simulink model "HostSerial_Receive"  (R2023b)
settings: Solver=FixedStepAuto  StartTime=0.0  StopTime=inf  FixedStep=0.001  RelTol=1e-3
libraries: instrumentseriallib x2
settings Model: Creator=ADMIN  LastModifiedBy=ADMIN
settings DataIOCC: ReturnWorkspaceOutputs=off
settings DebuggingCC: ParameterPrecisionLossMsg=none

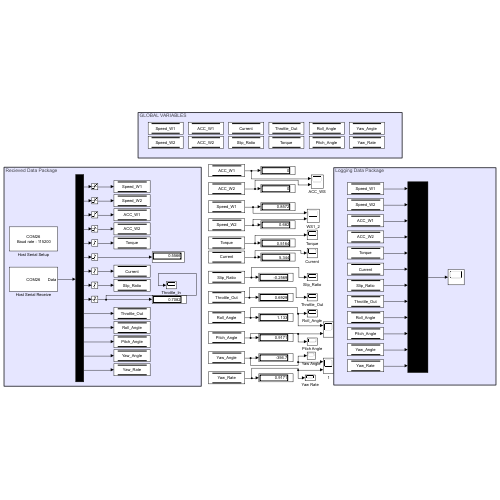
[thumbnail: Simulink's stored preview of the top-level diagram]
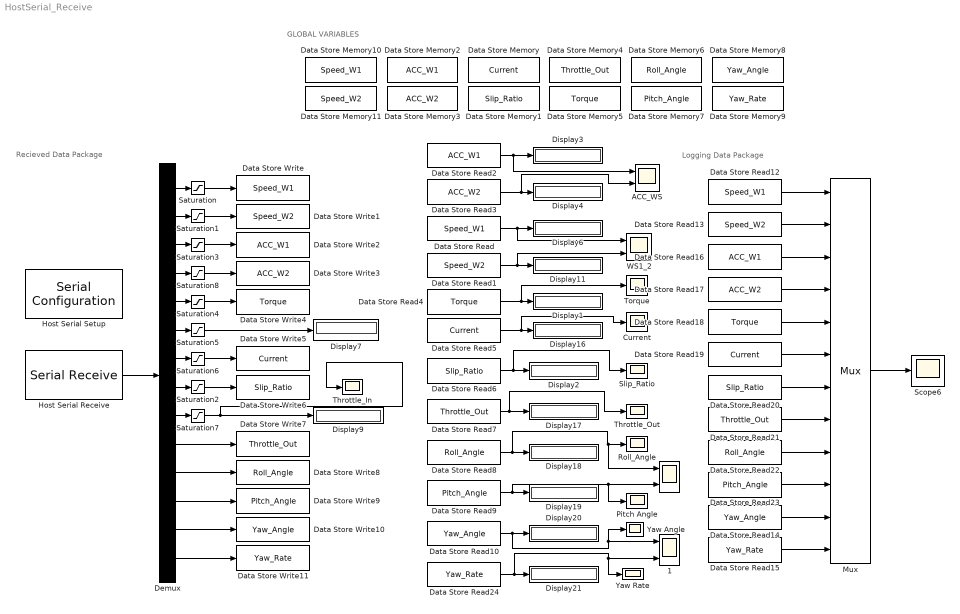
== system HostSerial_Receive ==
  note: Recieved Data Package
  note: Logging Data Package
  note: GLOBAL VARIABLES
  " " : Scope  NumInputPorts=2
  " 1" : Scope  NumInputPorts=2
  ACC_WS : Scope  NumInputPorts=2
  Current : Scope
  Data Store Memory : DataStoreMemory  DataStoreName=Current  WriteAfterWriteMsg=warning  ShowAdditionalParam=off  OutDataTypeStr=single
  Data Store Memory1 : DataStoreMemory  DataStoreName=Slip_Ratio  WriteAfterWriteMsg=warning  ShowAdditionalParam=off  OutDataTypeStr=single
  Data Store Memory10 : DataStoreMemory  DataStoreName=Speed_W1  WriteAfterWriteMsg=warning  ShowAdditionalParam=off  OutDataTypeStr=single
  Data Store Memory11 : DataStoreMemory  DataStoreName=Speed_W2  WriteAfterWriteMsg=warning  ShowAdditionalParam=off  OutDataTypeStr=single
  Data Store Memory2 : DataStoreMemory  DataStoreName=ACC_W1  WriteAfterWriteMsg=warning  ShowAdditionalParam=off  OutDataTypeStr=single
  Data Store Memory3 : DataStoreMemory  DataStoreName=ACC_W2  WriteAfterWriteMsg=warning  ShowAdditionalParam=off  OutDataTypeStr=single
  Data Store Memory4 : DataStoreMemory  DataStoreName=Throttle_Out  WriteAfterWriteMsg=warning  ShowAdditionalParam=off  OutDataTypeStr=single
  Data Store Memory5 : DataStoreMemory  DataStoreName=Torque  WriteAfterWriteMsg=warning  ShowAdditionalParam=off  OutDataTypeStr=single
  Data Store Memory6 : DataStoreMemory  DataStoreName=Roll_Angle  WriteAfterWriteMsg=warning  ShowAdditionalParam=off  OutDataTypeStr=single
  Data Store Memory7 : DataStoreMemory  DataStoreName=Pitch_Angle  WriteAfterWriteMsg=warning  ShowAdditionalParam=off  OutDataTypeStr=single
  Data Store Memory8 : DataStoreMemory  DataStoreName=Yaw_Angle  WriteAfterWriteMsg=warning  ShowAdditionalParam=off  OutDataTypeStr=single
  Data Store Memory9 : DataStoreMemory  DataStoreName=Yaw_Rate  WriteAfterWriteMsg=warning  ShowAdditionalParam=off  OutDataTypeStr=single
  Data Store Read : DataStoreRead  DataStoreName=Speed_W1  IndexOptions=Index vector (dialog)  Indices=1  OutputSizes=1
  Data Store Read1 : DataStoreRead  DataStoreName=Speed_W2  IndexOptions=Index vector (dialog)  Indices=1  OutputSizes=1
  Data Store Read10 : DataStoreRead  DataStoreName=Yaw_Angle  IndexOptions=Index vector (dialog)  Indices=1  OutputSizes=1
  Data Store Read12 : DataStoreRead  DataStoreName=Speed_W1  IndexOptions=Index vector (dialog)  Indices=1  OutputSizes=1
  Data Store Read13 : DataStoreRead  DataStoreName=Speed_W2  IndexOptions=Index vector (dialog)  Indices=1  OutputSizes=1
  Data Store Read14 : DataStoreRead  DataStoreName=Yaw_Angle  IndexOptions=Index vector (dialog)  Indices=1  OutputSizes=1
  Data Store Read15 : DataStoreRead  DataStoreName=Yaw_Rate  IndexOptions=Index vector (dialog)  Indices=1  OutputSizes=1
  Data Store Read16 : DataStoreRead  DataStoreName=ACC_W1  IndexOptions=Index vector (dialog)  Indices=1  OutputSizes=1
  Data Store Read17 : DataStoreRead  DataStoreName=ACC_W2  IndexOptions=Index vector (dialog)  Indices=1  OutputSizes=1
  Data Store Read18 : DataStoreRead  DataStoreName=Torque  IndexOptions=Index vector (dialog)  Indices=1  OutputSizes=1
  Data Store Read19 : DataStoreRead  DataStoreName=Current  IndexOptions=Index vector (dialog)  Indices=1  OutputSizes=1
  Data Store Read2 : DataStoreRead  DataStoreName=ACC_W1  IndexOptions=Index vector (dialog)  Indices=1  OutputSizes=1
  Data Store Read20 : DataStoreRead  DataStoreName=Slip_Ratio  IndexOptions=Index vector (dialog)  Indices=1  OutputSizes=1
  Data Store Read21 : DataStoreRead  DataStoreName=Throttle_Out  IndexOptions=Index vector (dialog)  Indices=1  OutputSizes=1
  Data Store Read22 : DataStoreRead  DataStoreName=Roll_Angle  IndexOptions=Index vector (dialog)  Indices=1  OutputSizes=1
  Data Store Read23 : DataStoreRead  DataStoreName=Pitch_Angle  IndexOptions=Index vector (dialog)  Indices=1  OutputSizes=1
  Data Store Read24 : DataStoreRead  DataStoreName=Yaw_Rate  IndexOptions=Index vector (dialog)  Indices=1  OutputSizes=1
  Data Store Read3 : DataStoreRead  DataStoreName=ACC_W2  IndexOptions=Index vector (dialog)  Indices=1  OutputSizes=1
  Data Store Read4 : DataStoreRead  DataStoreName=Torque  IndexOptions=Index vector (dialog)  Indices=1  OutputSizes=1
  Data Store Read5 : DataStoreRead  DataStoreName=Current  IndexOptions=Index vector (dialog)  Indices=1  OutputSizes=1
  Data Store Read6 : DataStoreRead  DataStoreName=Slip_Ratio  IndexOptions=Index vector (dialog)  Indices=1  OutputSizes=1
  Data Store Read7 : DataStoreRead  DataStoreName=Throttle_Out  IndexOptions=Index vector (dialog)  Indices=1  OutputSizes=1
  Data Store Read8 : DataStoreRead  DataStoreName=Roll_Angle  IndexOptions=Index vector (dialog)  Indices=1  OutputSizes=1
  Data Store Read9 : DataStoreRead  DataStoreName=Pitch_Angle  IndexOptions=Index vector (dialog)  Indices=1  OutputSizes=1
  Data Store Write : DataStoreWrite  DataStoreName=Speed_W1  IndexOptions=Index vector (dialog)  Indices=1  OutputSizes=1
  Data Store Write1 : DataStoreWrite  DataStoreName=Speed_W2  IndexOptions=Index vector (dialog)  Indices=1  OutputSizes=1
  Data Store Write10 : DataStoreWrite  DataStoreName=Yaw_Angle  IndexOptions=Index vector (dialog)  Indices=1  OutputSizes=1
  Data Store Write11 : DataStoreWrite  DataStoreName=Yaw_Rate  IndexOptions=Index vector (dialog)  Indices=1  OutputSizes=1
  Data Store Write2 : DataStoreWrite  DataStoreName=ACC_W1  IndexOptions=Index vector (dialog)  Indices=1  OutputSizes=1
  Data Store Write3 : DataStoreWrite  DataStoreName=ACC_W2  IndexOptions=Index vector (dialog)  Indices=1  OutputSizes=1
  Data Store Write4 : DataStoreWrite  DataStoreName=Torque  IndexOptions=Index vector (dialog)  Indices=1  OutputSizes=1
  Data Store Write5 : DataStoreWrite  DataStoreName=Current  IndexOptions=Index vector (dialog)  Indices=1  OutputSizes=1
  Data Store Write6 : DataStoreWrite  DataStoreName=Slip_Ratio  IndexOptions=Index vector (dialog)  Indices=1  OutputSizes=1
  Data Store Write7 : DataStoreWrite  DataStoreName=Throttle_Out  IndexOptions=Index vector (dialog)  Indices=1  OutputSizes=1
  Data Store Write8 : DataStoreWrite  DataStoreName=Roll_Angle  IndexOptions=Index vector (dialog)  Indices=1  OutputSizes=1
  Data Store Write9 : DataStoreWrite  DataStoreName=Pitch_Angle  IndexOptions=Index vector (dialog)  Indices=1  OutputSizes=1
  Demux : Demux  Outputs=14
  Display{1..4,6..7,9,11,16..21} (14 alike) : Display
  Host Serial Receive : instrumentseriallib/Serial Receive  PortSel=COM26  Port=COM26  ComPort=COM26  DataType=single  SaveDataType=uint8  ToggleHeader=on  Header=0xAA  ToggleTerminator=on  Terminator=Custom terminator  CustomTerminator=0xFF  InputFormat=Row major  ToggleDataSize=on  DataSize=14  EnableBlockingMode=on  ActionDataUnavailable=Output last received value  ActionWhenDataUnavailable=Output last received value  CustomValue=0  SampleTime=-1  SimulateUsing=Interpreted execution  BlockInModel=on  aMode=5
      settings: LibrarySourceBlock=mcblib/Protection and Diagnostics/Host Serial Receive
  Host Serial Setup : instrumentseriallib/Serial Configuration  Priority=-99  PortSel=COM26  Port=COM26  ComPort=COM26  BaudRate=115200  DataBits=8  Parity=none  StopBits=1  ByteOrder=little-endian  FlowControl=none  Timeout=1.0  SimulateUsing=Interpreted execution  BlockInModel=on  aMode=5
      settings: LibrarySourceBlock=mcblib/Protection and Diagnostics/Host Serial Setup
  Mux : Mux  Inputs=12
  Pitch Angle : Scope
  Roll_Angle : Scope
  Saturation : Saturate  UpperLimit=50  LowerLimit=0
  Saturation1 : Saturate  UpperLimit=50  LowerLimit=0
  Saturation2 : Saturate  UpperLimit=1  LowerLimit=-1
  Saturation3 : Saturate  UpperLimit=300  LowerLimit=-300
  Saturation4 : Saturate  UpperLimit=200  LowerLimit=0
  Saturation5 : Saturate  UpperLimit=250  LowerLimit=-250
  Saturation6 : Saturate  UpperLimit=200  LowerLimit=0
  Saturation7 : Saturate  UpperLimit=3.3  LowerLimit=0
  Saturation8 : Saturate  UpperLimit=300  LowerLimit=-300
  Scope6 : Scope
  Slip_Ratio : Scope
  Throttle_In : Scope
  Throttle_Out : Scope
  Torque : Scope
  WS1_2 : Scope  NumInputPorts=2
  Yaw Angle : Scope
  Yaw Rate : Scope
  wires:
  Host Serial Receive/1 -> Demux/1
  Demux/1 -> Saturation/1
  Demux/2 -> Saturation1/1
  Demux/6 -> Saturation5/1
  Demux/5 -> Saturation4/1
  Mux/1 -> Scope6/1
  Demux/9 -> Saturation7/1
  Saturation/1 -> Data Store Write/1
  Saturation1/1 -> Data Store Write1/1
  Saturation5/1 -> Display7/1
  Demux/7 -> Saturation6/1
  Saturation7/1 -> Display9/1, Throttle_In/1
  Demux/3 -> Saturation3/1
  Demux/4 -> Saturation8/1
  Saturation4/1 -> Data Store Write4/1
  Saturation6/1 -> Data Store Write5/1
  Demux/8 -> Saturation2/1
  Saturation2/1 -> Data Store Write6/1
  Demux/10 -> Data Store Write7/1
  Demux/11 -> Data Store Write8/1
  Demux/12 -> Data Store Write9/1
  Demux/13 -> Data Store Write10/1
  Demux/14 -> Data Store Write11/1
  Data Store Read12/1 -> Mux/1
  Data Store Read13/1 -> Mux/2
  Data Store Read16/1 -> Mux/3
  Data Store Read17/1 -> Mux/4
  Data Store Read18/1 -> Mux/5
  Data Store Read19/1 -> Mux/6
  Data Store Read15/1 -> Mux/12
  Data Store Read14/1 -> Mux/11
  Data Store Read23/1 -> Mux/10
  Data Store Read22/1 -> Mux/9
  Data Store Read21/1 -> Mux/8
  Data Store Read20/1 -> Mux/7
  Data Store Read3/1 -> ACC_WS/2, Display4/1
  Data Store Read2/1 -> Display3/1, ACC_WS/1
  Data Store Read/1 -> WS1_2/1, Display6/1
  Data Store Read1/1 -> WS1_2/2, Display11/1
  Data Store Read4/1 -> Torque/1, Display1/1
  Data Store Read5/1 -> Current/1, Display16/1
  Data Store Read6/1 -> Slip_Ratio/1, Display2/1
  Data Store Read7/1 -> Throttle_Out/1, Display17/1
  Data Store Read9/1 -> " "/2, Pitch Angle/1, Display19/1
  Data Store Read8/1 -> " "/1, Roll_Angle/1, Display18/1
  Data Store Read10/1 -> Yaw Angle/1, " 1"/1, Display20/1
  Data Store Read24/1 -> Yaw Rate/1, " 1"/2, Display21/1
  Saturation3/1 -> Data Store Write2/1
  Saturation8/1 -> Data Store Write3/1
